simulink model "sampleModel1653"  (R2023a)
settings: Solver=VariableStepAuto  StartTime=0.0  StopTime=10.0  RelTol=1e-3
libraries: simulink x3, hdlsllib x3
settings Model: Creator=user1  LastModifiedBy=user1

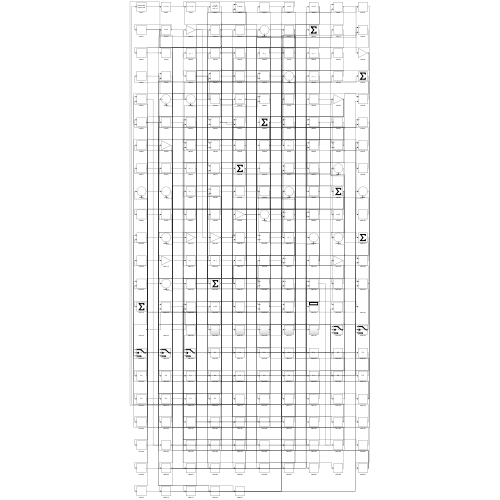
[thumbnail: Simulink's stored preview of the top-level diagram]
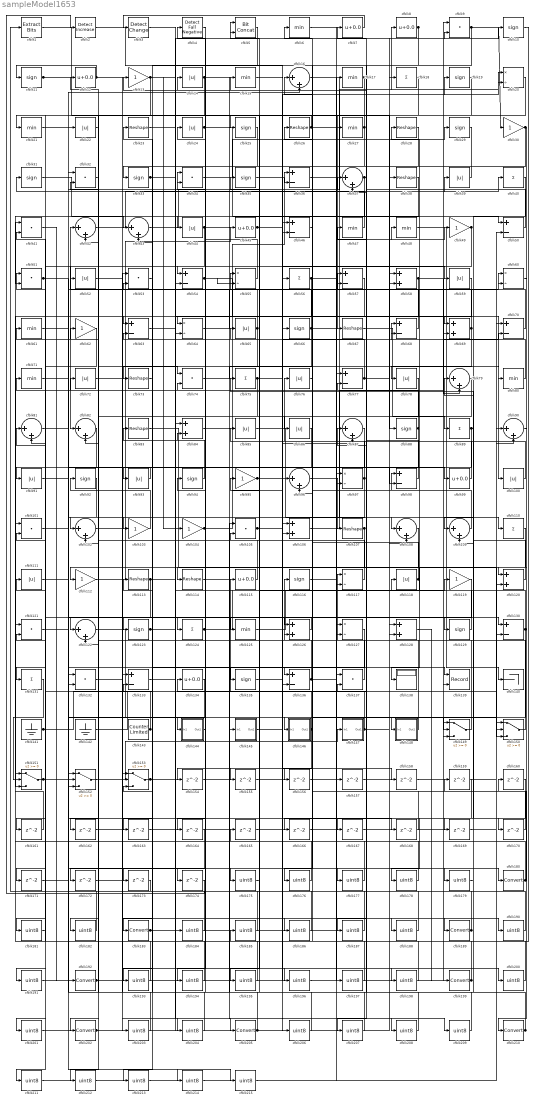
== system sampleModel1653 ==
  cfblk1 : simulink/Logic and Bit Operations/Extract Bits  bitsToExtract=Upper half  numBits=8  bitIdxRange=[0 7]  outScalingMode=Preserve fixed-point scaling
      settings: LibrarySourceBlock=|
      | hdlsllib/Logic and Bit
      | Operations/Extract Bits
  cfblk{10..11,19,25,29,31,33,35,66,88,92,94,116,123,129,135} (16 alike) : Signum
  cfblk{14,22,24,39,44,52,59,65,72,76,78,85..86,91,93,100,111,118} (18 alike) : Abs  SaturateOnIntegerOverflow=off
  cfblk{9,32,34,41,51,53,74,101,105,121,132,137} (12 alike) : DotProduct  OutDataTypeStr=Inherit: Inherit via internal rule
  cfblk{16,37,42..43,79,81..82,87,90,96,102,108..109,122} (14 alike) : Sum  Inputs=|++
  cfblk{13,30,49,62,95,103..104,112,119} (9 alike) : Gain
  cfblk{58,69,84,106,120,126,128} (7 alike) : Sum
  cfblk{23,26,28,38,67,73,83,107,113..114} (10 alike) : Reshape
  cfblk{18,40,56,75,89,110,124,131} (8 alike) : Sum  Inputs=+
  cfblk{7..8,12,45,99,115,134} (7 alike) : Bias  Bias=0.0  SaturateOnIntegerOverflow=off
  cfblk{20,55,60,64,97,117,127} (7 alike) : Product  Inputs=*/  RndMeth=Zero  SaturateOnIntegerOverflow=on
  cfblk{6,15,17,21,27,47..48,61,71,80,125} (11 alike) : MinMax
  cfblk{36,46,50,54,57,63,68,70,77,98,130,133,136} (13 alike) : Sum  Inputs=+-
  cfblk138 : Display
  cfblk139 : Record  FileSettingsInternal="{\"entries\":[{\"content\":{\"excelSettings\":{\"content\":{},\"type\":\"Streamout.ExcelSettings\"}},\"type\":\"Streamout.FileSettingStorage\",\"uuid\":\"\"}],\"packageUris\":[\"http:\\/\\/schema.mathworks.com\\/mf0\\/streamout_blocks\\/R2020a\"],\"version\":\"1.0\"}"  Layout=[1 1]  SignalsInternal="{\"entries\":[{\"content\":{\"signals\":[{\"content\":{\"blockPath\":[],\"dimensions\":[1],\"domain\":\"\",\"lineColor\":\"#a2142f\",\"plots\":[1],\"port\":1,\"signalID\":2556,\"signalName\":\"XY Graph:1\"},\"type\":\"RecordBlkView.Signal\",\"uuid\":\"\"},{\"content\":{\"blockPath\":[],\"dimensions\":[1],\"domain\":\"\",\"lineColor\":\"#139fff\",\"plots\":[1],\"port\":2,\"signalID\":2559,\"signalName\":\"XY Graph:2\"},\"type\":\"RecordBlkView.Signal\",\"uuid\":\"\"}]},\"type\":\"RecordBlkView.InputSignals\",\"uuid\":\"\"}],\"packageUris\":[\"http:\\/\\/schema.mathworks.com\\/mf0\\/streamout_blocks\\/R2020a\"],\"version\":\"1.0\"}"  VisualizationBindings="{\"xyplotplugin\":{\"info\":[{\"series\":[{\"bindingParametersList\":[{\"parameter\":\"X-Axis\",\"signalID\":2556,\"signalName\":\"XY Graph:1\"},{\"parameter\":\"Y-Axis\",\"signalID\":2559,\"signalName\":\"XY Graph:2\"}],\"seriesID\":63475}],\"subplotID\":1}]}}"  CompatibilityTag=XY  st=-1
  cfblk140 : Terminator
  cfblk141 : Ground
  cfblk142 : Ground
  cfblk143 : hdlsllib/Sources/Counter Limited  uplimit=7  tsamp=-1
  cfblk144 : Subsystem
      settings: LibrarySourceBlock=|
      | hdlsllib/Ports &
      | Subsystems/Subsystem
  cfblk145 : Subsystem
      settings: LibrarySourceBlock=|
      | hdlsllib/Ports &
      | Subsystems/Subsystem
  cfblk146 : Subsystem
      settings: LibrarySourceBlock=|
      | hdlsllib/Ports &
      | Subsystems/Subsystem
  cfblk147 : Subsystem
      settings: LibrarySourceBlock=|
      | hdlsllib/Ports &
      | Subsystems/Subsystem
  cfblk148 : Subsystem
      settings: LibrarySourceBlock=|
      | hdlsllib/Ports &
      | Subsystems/Subsystem
  cfblk{149..153} (5 alike) : Switch  SaturateOnIntegerOverflow=off  InputSameDT=off
  cfblk{154..174} (21 alike) : Delay  SampleTime=1
  cfblk{175..179,181..182,184..188,190..191,193..198,200..201,203..204,206..209,211..215} (33 alike) : DataTypeConversion  OutDataTypeStr=uint8  SaturateOnIntegerOverflow=off  RndMeth=Floor
  cfblk{180,183,189,192,199,202,205,210} (8 alike) : DataTypeConversion  SaturateOnIntegerOverflow=off  RndMeth=Floor
  cfblk2 : simulink/Logic and Bit Operations/Detect Increase  vinit=0.0  OutDataTypeStr=boolean
      settings: LibrarySourceBlock=|
      | hdlsllib/Logic and Bit
      | Operations/Detect
      | Increase
  cfblk3 : simulink/Logic and Bit Operations/Detect Change  vinit=0  OutDataTypeStr=boolean
      settings: LibrarySourceBlock=|
      | hdlsllib/Logic and Bit
      | Operations/Detect
      | Change
  cfblk4 : hdlsllib/Logic and Bit Operations/Detect Fall Negative  vinit=0  OutDataTypeStr=boolean
  cfblk5 : hdlsllib/Logic and Bit Operations/Bit Concat  numInputs=2
  wires:
  cfblk112/1 -> cfblk45/1
  cfblk94/1 -> cfblk83/1
  cfblk104/1 -> cfblk36/1, cfblk20/2
  cfblk122/1 -> cfblk144/1(In1)
  cfblk118/1 -> cfblk26/1, cfblk98/1
  cfblk21/1 -> cfblk22/1
  cfblk131/1 -> cfblk151/2
  cfblk12/1 -> cfblk11/1, cfblk74/1
  cfblk34/1 -> cfblk29/1
  cfblk42/1 -> cfblk39/1
  cfblk48/1 -> cfblk140/1
  cfblk93/1 -> cfblk91/1
  cfblk44/1 -> cfblk82/1, cfblk69/1, cfblk209/1
  cfblk95/1 -> cfblk114/1, cfblk87/2, cfblk149/2
  cfblk120/1 -> cfblk75/1
  cfblk16/1 -> cfblk108/1
  cfblk20/1 -> cfblk67/1
  cfblk53/1 -> cfblk183/1
  cfblk103/1 -> cfblk72/1
  cfblk26/1 -> cfblk21/1, cfblk20/1
  cfblk147/1(Out1) -> cfblk115/1, cfblk10/1
  cfblk124/1 -> cfblk17/1, cfblk118/1
  cfblk15/1 -> cfblk50/1
  cfblk117/1 -> cfblk65/1
  cfblk107/1 -> cfblk122/1, cfblk155/1
  cfblk146/1(Out1) -> cfblk34/1, cfblk164/1
  cfblk55/1 -> cfblk4/1
  cfblk24/1 -> cfblk56/1, cfblk98/2
  cfblk129/1 -> cfblk28/1
  cfblk137/1 -> cfblk117/1
  cfblk19/1 -> cfblk93/1
  cfblk81/1 -> cfblk180/1
  cfblk36/1 -> cfblk100/1
  cfblk67/1 -> cfblk89/1
  cfblk151/1 -> cfblk60/2, cfblk214/1
  cfblk83/1 -> cfblk150/2
  cfblk98/1 -> cfblk13/1
  cfblk2/1 -> cfblk66/1
  cfblk113/1 -> cfblk146/1(In1), cfblk153/2
  cfblk65/1 -> cfblk42/1, cfblk172/1
  cfblk133/1 -> cfblk205/1
  cfblk40/1 -> cfblk109/1
  cfblk128/1 -> cfblk199/1
  cfblk37/1 -> cfblk51/2, cfblk167/1
  cfblk132/1 -> cfblk189/1
  cfblk30/1 -> cfblk120/1, cfblk97/2
  cfblk115/1 -> cfblk61/1
  cfblk54/1 -> cfblk24/1, cfblk106/1, cfblk55/2
  cfblk4/1 -> cfblk64/1
  cfblk136/1 -> cfblk116/1, cfblk179/1
  cfblk89/1 -> cfblk122/2, cfblk136/2, cfblk169/1
  cfblk7/1 -> cfblk3/1
  cfblk61/1 -> cfblk99/1
  cfblk35/1 -> cfblk36/2
  cfblk153/1 -> cfblk38/1, cfblk139/2
  cfblk11/1 -> cfblk145/1(In1), cfblk117/2
  cfblk125/1 -> cfblk77/1
  cfblk17/1 -> cfblk102/1, cfblk57/2
  cfblk59/1 -> cfblk64/2
  cfblk126/1 -> cfblk123/1
  cfblk100/1 -> cfblk57/1
  cfblk149/1 -> cfblk23/1
  cfblk87/1 -> cfblk102/2
  cfblk27/1 -> cfblk25/1, cfblk73/1
  cfblk101/1 -> cfblk135/1
  cfblk25/1 -> cfblk124/1
  cfblk43/1 -> cfblk8/1
  cfblk71/1 -> cfblk130/1
  cfblk109/1 -> cfblk15/1
  cfblk99/1 -> cfblk85/1
  cfblk22/1 -> cfblk42/2
  cfblk78/1 -> cfblk82/2
  cfblk123/1 -> cfblk9/2, cfblk119/1
  cfblk69/1 -> cfblk78/1, cfblk47/1, cfblk43/2
  cfblk56/1 -> cfblk48/1, cfblk106/2, cfblk194/1
  cfblk105/1 -> cfblk5/1, cfblk68/2
  cfblk50/1 -> cfblk14/1
  cfblk148/1(Out1) -> cfblk7/1
  cfblk1/1 -> cfblk88/1
  cfblk85/1 -> cfblk110/1
  cfblk80/1 -> cfblk68/1
  cfblk92/1 -> cfblk152/2
  cfblk8/1 -> cfblk166/1, cfblk187/1
  cfblk75/1 -> cfblk19/1, cfblk154/1
  cfblk3/1 -> cfblk139/1
  cfblk97/1 -> cfblk76/1, cfblk182/1
  cfblk68/1 -> cfblk35/1
  cfblk106/1 -> cfblk70/2
  cfblk90/1 -> cfblk210/1
  cfblk96/1 -> cfblk107/1
  cfblk62/1 -> cfblk131/1
  cfblk91/1 -> cfblk16/2
  cfblk58/1 -> cfblk79/2, cfblk151/3
  cfblk39/1 -> cfblk33/1
  cfblk45/1 -> cfblk59/1, cfblk177/1
  cfblk79/1 -> cfblk112/1
  cfblk13/1 -> cfblk104/1, cfblk69/2, cfblk181/1
  cfblk111/1 -> cfblk37/1
  cfblk142/1 -> cfblk130/2
  cfblk31/1 -> cfblk43/1
  cfblk152/1 -> cfblk147/1(In1)
  cfblk110/1 -> cfblk138/1
  cfblk76/1 -> cfblk136/1
  cfblk108/1 -> cfblk125/1
  cfblk66/1 -> cfblk40/1, cfblk55/1, cfblk174/1
  cfblk9/1 -> cfblk30/1, cfblk63/1
  cfblk51/1 -> cfblk148/1(In1), cfblk168/1
  cfblk74/1 -> cfblk80/1
  cfblk141/1 -> cfblk96/1, cfblk101/2, cfblk191/1
  cfblk134/1 -> cfblk152/3
  cfblk32/1 -> cfblk202/1
  cfblk64/1 -> cfblk60/1
  cfblk41/1 -> cfblk192/1
  cfblk23/1 -> cfblk150/3
  cfblk47/1 -> cfblk31/1
  cfblk143/1 -> cfblk111/1, cfblk51/1
  cfblk150/1 -> cfblk71/1
  cfblk14/1 -> cfblk52/1, cfblk196/1
  cfblk77/1 -> cfblk49/1, cfblk63/2
  cfblk5/1 -> cfblk44/1
  cfblk130/1 -> cfblk105/2, cfblk156/1
  cfblk70/1 -> cfblk37/2
  cfblk33/1 -> cfblk126/1, cfblk129/1
  cfblk46/1 -> cfblk96/2
  cfblk144/1(Out1) -> cfblk94/1
  cfblk88/1 -> cfblk103/1, cfblk12/1
  cfblk49/1 -> cfblk86/1, cfblk54/1, cfblk201/1
  cfblk154/1 -> cfblk120/2
  cfblk155/1 -> cfblk46/1
  cfblk156/1 -> cfblk108/2
  cfblk157/1 -> cfblk150/1
  cfblk135/1 -> cfblk158/1
  cfblk158/1 -> cfblk9/1
  cfblk57/1 -> cfblk161/1
  cfblk161/1 -> cfblk151/1
  cfblk38/1 -> cfblk162/1
  cfblk162/1 -> cfblk58/1
  cfblk29/1 -> cfblk163/1
  cfblk163/1 -> cfblk50/2
  cfblk166/1 -> cfblk126/2
  cfblk167/1 -> cfblk70/1
  cfblk168/1 -> cfblk77/2
  cfblk169/1 -> cfblk79/1
  cfblk60/1 -> cfblk170/1
  cfblk170/1 -> cfblk16/1
  cfblk119/1 -> cfblk171/1
  cfblk73/1 -> cfblk173/1
  cfblk173/1 -> cfblk1/1
  cfblk174/1 -> cfblk2/1
  cfblk121/1 -> cfblk175/1
  cfblk175/1 -> cfblk95/1
  cfblk160/1 -> cfblk176/1
  cfblk176/1 -> cfblk121/1
  cfblk177/1 -> cfblk121/2
  cfblk159/1 -> cfblk178/1
  cfblk178/1 -> cfblk137/2
  cfblk179/1 -> cfblk159/1
  cfblk180/1 -> cfblk160/1, cfblk153/3, cfblk74/2
  cfblk181/1 -> cfblk81/1
  cfblk182/1 -> cfblk81/2
  cfblk183/1 -> cfblk157/1, cfblk97/1
  cfblk63/1 -> cfblk184/1
  cfblk184/1 -> cfblk53/1
  cfblk10/1 -> cfblk185/1
  cfblk185/1 -> cfblk53/2
  cfblk84/1 -> cfblk186/1
  cfblk186/1 -> cfblk101/1
  cfblk187/1 -> cfblk84/1
  cfblk116/1 -> cfblk188/1
  cfblk188/1 -> cfblk84/2
  cfblk189/1 -> cfblk149/1, cfblk62/1
  cfblk114/1 -> cfblk190/1
  cfblk190/1 -> cfblk132/1
  cfblk191/1 -> cfblk132/2
  cfblk192/1 -> cfblk149/3, cfblk46/2
  cfblk86/1 -> cfblk193/1
  cfblk193/1 -> cfblk41/1
  cfblk194/1 -> cfblk41/2
  cfblk18/1 -> cfblk195/1
  cfblk195/1 -> cfblk152/1
  cfblk196/1 -> cfblk18/1
  cfblk6/1 -> cfblk197/1
  cfblk197/1 -> cfblk92/1
  cfblk102/1 -> cfblk198/1
  cfblk198/1 -> cfblk6/1
  cfblk199/1 -> cfblk153/1, cfblk113/1
  cfblk52/1 -> cfblk200/1
  cfblk200/1 -> cfblk128/1
  cfblk201/1 -> cfblk128/2
  cfblk202/1 -> cfblk54/2, cfblk27/1, cfblk58/2
  cfblk72/1 -> cfblk203/1
  cfblk203/1 -> cfblk32/1
  cfblk172/1 -> cfblk204/1
  cfblk204/1 -> cfblk32/2
  cfblk205/1 -> cfblk105/1, cfblk34/2
  cfblk145/1(Out1) -> cfblk206/1
  cfblk206/1 -> cfblk133/1
  cfblk28/1 -> cfblk207/1
  cfblk207/1 -> cfblk133/2
  cfblk165/1 -> cfblk208/1
  cfblk208/1 -> cfblk5/2
  cfblk209/1 -> cfblk165/1
  cfblk210/1 -> cfblk134/1, cfblk109/2, cfblk87/1
  cfblk82/1 -> cfblk211/1
  cfblk211/1 -> cfblk90/1
  cfblk164/1 -> cfblk212/1
  cfblk212/1 -> cfblk90/2
  cfblk127/1 -> cfblk213/1
  cfblk213/1 -> cfblk137/1
  cfblk214/1 -> cfblk127/1
  cfblk171/1 -> cfblk215/1
  cfblk215/1 -> cfblk127/2

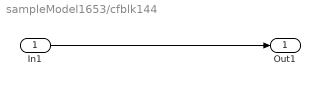
== system sampleModel1653/cfblk144 ==
  In1 : Inport
  Out1 : Outport
  wires:
  In1/1 -> Out1/1

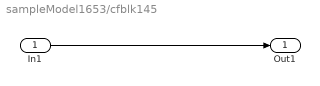
== system sampleModel1653/cfblk145 ==
  In1 : Inport
  Out1 : Outport
  wires:
  In1/1 -> Out1/1

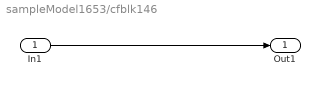
== system sampleModel1653/cfblk146 ==
  In1 : Inport
  Out1 : Outport
  wires:
  In1/1 -> Out1/1

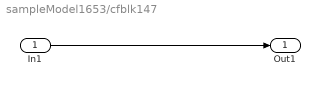
== system sampleModel1653/cfblk147 ==
  In1 : Inport
  Out1 : Outport
  wires:
  In1/1 -> Out1/1

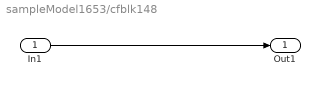
== system sampleModel1653/cfblk148 ==
  In1 : Inport
  Out1 : Outport
  wires:
  In1/1 -> Out1/1
